simulink model "ports1"  (R2014a)
settings: Solver=ode45  StartTime=0.0  StopTime=10.0  RelTol=1e-3
settings Model: Creator=ladmin  LastModifiedBy=ladmin

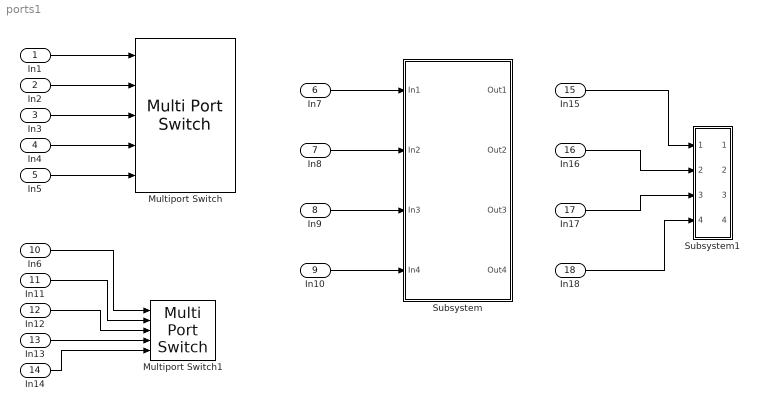
== system ports1 ==
  In1 : Inport
  In2 : Inport  Port=2
  In3 : Inport  Port=3
  In4 : Inport  Port=4
  In5 : Inport  Port=5
  In7 : Inport  Port=6
  In8 : Inport  Port=7
  In9 : Inport  Port=8
  In10 : Inport  Port=9
  In6 : Inport  Port=10
  In11 : Inport  Port=11
  In12 : Inport  Port=12
  In13 : Inport  Port=13
  In14 : Inport  Port=14
  In15 : Inport  Port=15
  In16 : Inport  Port=16
  In17 : Inport  Port=17
  In18 : Inport  Port=18
  Multiport Switch : MultiPortSwitch  Inputs=4
  Multiport Switch1 : MultiPortSwitch  Inputs=4
  Subsystem : Subsystem
  Subsystem1 : Subsystem
  wires:
  In5/1 -> Multiport Switch/5
  In4/1 -> Multiport Switch/4
  In3/1 -> Multiport Switch/3
  In2/1 -> Multiport Switch/2
  In1/1 -> Multiport Switch/1
  In7/1 -> Subsystem/1(In1)
  In8/1 -> Subsystem/2(In2)
  In9/1 -> Subsystem/3(In3)
  In10/1 -> Subsystem/4(In4)
  In14/1 -> Multiport Switch1/5
  In13/1 -> Multiport Switch1/4
  In12/1 -> Multiport Switch1/3
  In11/1 -> Multiport Switch1/2
  In6/1 -> Multiport Switch1/1
  In15/1 -> Subsystem1/1(In1)
  In16/1 -> Subsystem1/2(In2)
  In17/1 -> Subsystem1/3(In3)
  In18/1 -> Subsystem1/4(In4)

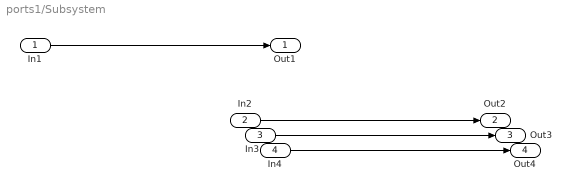
== system ports1/Subsystem ==
  In1 : Inport
  In2 : Inport  Port=2
  In3 : Inport  Port=3
  In4 : Inport  Port=4
  Out1 : Outport
  Out2 : Outport  Port=2
  Out3 : Outport  Port=3
  Out4 : Outport  Port=4
  wires:
  In1/1 -> Out1/1
  In2/1 -> Out2/1
  In3/1 -> Out3/1
  In4/1 -> Out4/1

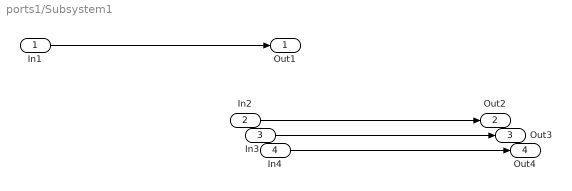
== system ports1/Subsystem1 ==
  In1 : Inport
  In2 : Inport  Port=2
  In3 : Inport  Port=3
  In4 : Inport  Port=4
  Out1 : Outport
  Out2 : Outport  Port=2
  Out3 : Outport  Port=3
  Out4 : Outport  Port=4
  wires:
  In1/1 -> Out1/1
  In2/1 -> Out2/1
  In3/1 -> Out3/1
  In4/1 -> Out4/1
